simulink model "cv_mutual_exclusion"  (Simulink 6.0)
settings: Solver=ode45  StartTime=0.0  StopTime=10.0  RelTol=1e-3
settings Model: RecordCoverage=on  CovCompData=covdata  CovNameIncrementing=on  Creator=The MathWorks Inc.  LastModifiedBy=batserve  ExtModeAutoUpdateStatusClock=off  ProdHWDeviceType=Specified
settings DataIOCC: SignalLoggingName=logsOut
settings DebuggingCC: CheckExecutionContextPreStartOutputMsg=on  CheckExecutionContextRuntimeOutputMsg=on  SolverPrmCheckMsg=none
settings HardwareCC: ProdHWDeviceType=Specified

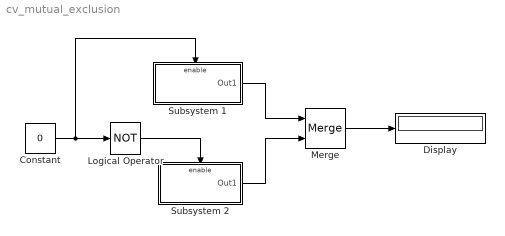
== system cv_mutual_exclusion ==
  Constant : Constant  Value=0
  Display : Display
  Logical Operator : Logic  Operator=NOT  AllPortsSameDT=off  OutDataTypeMode=Boolean
  Merge : Merge
  Subsystem 1 : Subsystem  PropExecContextAcrossSSBoundary=on
  Subsystem 2 : Subsystem  PropExecContextAcrossSSBoundary=on
  wires:
  Logical Operator/1 -> Subsystem 2/Enable
  Constant/1 -> Logical Operator/1, Subsystem 1/Enable
  Merge/1 -> Display/1
  Subsystem 2/1(Out1) -> Merge/2
  Subsystem 1/1(Out1) -> Merge/1

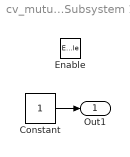
== system cv_mutual_exclusion/Subsystem 1 ==
  Enable : EnablePort
  Constant : Constant
  Out1 : Outport  InitialOutput=0
  wires:
  Constant/1 -> Out1/1

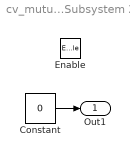
== system cv_mutual_exclusion/Subsystem 2 ==
  Enable : EnablePort
  Constant : Constant  Value=0
  Out1 : Outport  InitialOutput=0
  wires:
  Constant/1 -> Out1/1
